simulink model "px4demo_PWM_WITH_RC"  (R2018b)
settings: Solver=FixedStepAuto  StartTime=0.0  StopTime=inf  RelTol=1e-3  EnableMultiTasking=on
undefined symbols (not defined in the file or in its folder): dev, Main, pwm_output0
libraries: px4lib x1, px4Sensorslib x1
settings Model: SimulationMode=external  ExtModeTrigDuration=10  Creator=The MathWorks, Inc.  LastModifiedBy=Tejas Rajopadhye
settings SolverCC: PositivePriorityOrder=on
settings DataIOCC: ReturnWorkspaceOutputs=on
settings OptimizationCC: EnhancedBackFolding=on  PassReuseOutputArgsAs=Individual arguments  MaxStackSize=64  OptimizeBlockOrder=speed  DifferentSizesBufferReuse=on  OptimizationCustomize=off
settings DebuggingCC: ParameterTunabilityLossMsg=error
settings HardwareCC: ProdBitPerPointer=32  ProdBitPerSizeT=32  ProdBitPerPtrDiffT=32  ProdLargestAtomicInteger=Long  ProdLargestAtomicFloat=Double  ProdWordSize=32  ProdLongLongMode=on  ProdHWDeviceType=ARM Compatible->ARM Cortex
settings SFSimCC: MATLABDynamicMemAlloc=off
settings RTWCC: SystemTargetFile=ert.tlc  HardwareBoard=PX4 Pixhawk 4  TLCOptions="-aInlineSetEventsForThisBaseRateFcn=TLC_FALSE -aSuppressMultiTaskScheduler=TLC_FALSE  -aRateBasedStepFcn=0"  TemplateMakefile=ert_default_tmf  GenerateReport=on  Toolchain=GNU Tools for PX4 Autopilots  IncludeHyperlinkInReport=on  LaunchReport=on  TargetLang=C++  GenerateTraceInfo=on  GenerateTraceReport=on  GenerateTraceReportSl=on  GenerateTraceReportSf=on  GenerateTraceReportEml=on
settings CodeAppCC: ForceParamTrailComments=on  IgnoreCustomStorageClasses=off  OperatorAnnotations=on  SimulinkDataObjDesc=on  SFDataObjDesc=on  InsertBlockDesc=on

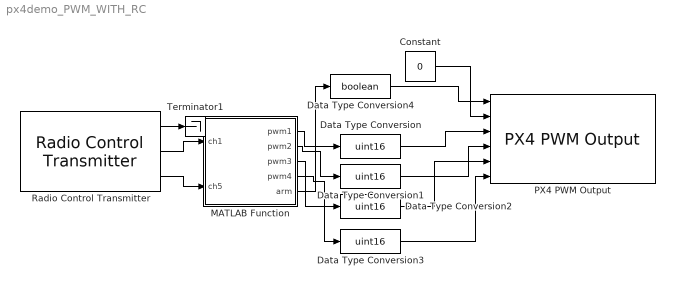
== system px4demo_PWM_WITH_RC ==
  Constant : Constant  Value=0  OutDataTypeStr=boolean
  Data Type Conversion{,1..3} (4 alike) : DataTypeConversion  OutDataTypeStr=uint16
  Data Type Conversion4 : DataTypeConversion  OutDataTypeStr=boolean
  MATLAB Function : MATLAB Function  TreatAsAtomicUnit=on
  PX4 PWM Output : px4lib/PX4 PWM Output  pwmDevice=Main (/dev/pwm_output0)  pwmChannel1_=on  pwmChannel2_=on  pwmChannel3_=on  pwmChannel4_=on  pwmChannel5_=off  pwmChannel6_=off  pwmChannel7_=off  pwmChannel8_=off  forceTerminateFailsafe=off  outputErrorStatus=off
      settings: SourceProductName=Embedded Coder Support Package for PX4 Autopilots  SourceProductBaseCode=PX4AUTOPILOTS
  Radio Control Transmitter : px4Sensorslib/Radio Control Transmitter  channel1=on  channel2=off  channel3=off  channel4=off  channel5=on  channel6=off  channel7=off  channel8=off  channel_count=off  rssi=off  rc_input_source=off  timestamp_last_signal=off  time_stamp=off  sampleTime=1/250  BlockingMode=off  BlockTimeout=5
      settings: SourceProductName=Embedded Coder Support Package for PX4 Autopilots
  Terminator1 : Terminator
  wires:
  Radio Control Transmitter/1 -> Terminator1/1
  Constant/1 -> PX4 PWM Output/2
  Radio Control Transmitter/2 -> MATLAB Function/1(ch1)
  MATLAB Function/1(pwm1) -> Data Type Conversion/1
  MATLAB Function/2(pwm2) -> Data Type Conversion1/1
  MATLAB Function/3(pwm3) -> Data Type Conversion2/1
  MATLAB Function/4(pwm4) -> Data Type Conversion3/1
  Data Type Conversion/1 -> PX4 PWM Output/3
  Data Type Conversion1/1 -> PX4 PWM Output/4
  Data Type Conversion2/1 -> PX4 PWM Output/5
  Data Type Conversion3/1 -> PX4 PWM Output/6
  Radio Control Transmitter/3 -> MATLAB Function/2(ch5)
  MATLAB Function/5(arm) -> Data Type Conversion4/1
  Data Type Conversion4/1 -> PX4 PWM Output/1

== matlab function px4demo_PWM_WITH_RC/MATLAB Function ==
  data: ch1 input; pwm1 output; pwm2 output; pwm3 output; pwm4 output; ch5 input; arm output
function [pwm1, pwm2, pwm3, pwm4, arm] = pwm_out(ch1, ch5)
pwm1 = ch1;
pwm2 = ch1;
pwm3 = ch1;
pwm4 = ch1;
if (ch5 > single(1500))
    arm = true;
else
    arm = false;
end
